simulink model "LongPRACH_sim"  (R2023b)
settings: Solver=FixedStepDiscrete  StartTime=0.0  StopTime=prach.SimulationTime  FixedStep=1  RelTol=1e-3  EnableMultiTasking=on
PreLoadFcn:
  | warning off Simulink:Commands:SetParamLinkChangeWarn
  | warning off Simulink:Commands:LoadMdlParameterizedLink
  | warning off Simulink:SL_SetParamLinkChangeWarn
  | warning off Simulink:SL_LoadMdlParameterizedLink
  | setup_LongPRACH;
InitFcn:
  | setup_LongPRACH;
StopFcn:
  | %prach_out_analysis;
  | prach_analysis
values from neighbouring files (symbols this model uses):
  prach = nrPRACHConfig('FrequencyRange','FR1','DuplexMode','TDD','ConfigurationIndex',config_idx,'SubcarrierSpacing',1.25,'SequenceIndex',ZCseq,          'PreambleIndex', cs_idx,'RBOffset',nRB,'ZeroCorrelationZone', N_cs, 'RestrictedSet','UnrestrictedSet', 'ActivePRACHSlot', 0 ,'FrequencyIndex', ii-1, 'TimeIndex',0,'NPRACHSlot',0)    [prach_gen_5g_toolbox.m]
undefined symbols (not defined in the file or in its folder): dpoly, value
libraries: DSPBAPrim x27, DSPBABase x7, dspsrcs4 x3, DSPBAUtilities x1, DSPBAControl x1, Lib_LongPRACH x1
Description:
  | This design example implements a long PRACH format-0 processing for NR - RU
settings Model: Creator=lrigby  LastModifiedBy=manjukri
settings SolverCC: AlgebraicLoopSolver=TrustRegion
settings DataIOCC: LimitDataPoints=on  SaveFormat=Array  SignalLoggingSaveFormat=ModelDataLogs  ReturnWorkspaceOutputs=off
settings OptimizationCC: ExpressionDepthLimit=2147483647  InitFltsAndDblsToZero=on  LifeSpan=inf
settings DebuggingCC: SaveWithParameterizedLinksMsg=none  UnderspecifiedInitializationDetection=Classic  MergeDetectMultiDrivingBlocksExec=none  SignalResolutionControl=TryResolveAllWithWarning  SolverPrmCheckMsg=warning  ParameterPrecisionLossMsg=none  UnconnectedInputMsg=warning  UnconnectedOutputMsg=warning  UnconnectedLineMsg=warning  StateNameClashWarn=warning  SFUnexpectedBacktrackingDiag=warning  SFNoUnconditionalDefaultTransitionDiag=warning  SFExecutionAtInitializationDiag=none  ArithmeticOperatorsInVariantConditions=warning
settings HardwareCC: ProdBitPerPointer=32  ProdBitPerSizeT=32  ProdBitPerPtrDiffT=32  ProdLargestAtomicFloat=None  ProdIntDivRoundTo=Undefined  ProdEndianess=Unspecified  ProdWordSize=32  ProdHWDeviceType=ASIC/FPGA  TargetBitPerLong=64  TargetBitPerPointer=64  TargetBitPerSizeT=64  TargetBitPerPtrDiffT=64  TargetLongLongMode=on  TargetIntDivRoundTo=Zero  TargetEndianess=LittleEndian  TargetWordSize=64  TargetHWDeviceType=MATLAB Host  ProdEqTarget=off
settings ModelReferenceCC: EnableRefExpFcnMdlSchedulingChecks=on  PropagateSignalLabelsOutOfModel=off
settings SFSimCC: SimUseLocalCustomCode=off  SimParseCustomCode=off  CustomCodeUndefinedFunction=UseInterfaceOnly
settings RTWCC: RTWUseLocalCustomCode=off  DLArmComputeVersion=19.05
settings CodeAppCC: StateflowObjectComments=on
settings GRTTargetCC: TargetFcnLib=ansi_tfl_tmw.mat  TargetLangStandard=C89/C90 (ANSI)  CombineOutputUpdateFcns=off  GRTInterface=on
settings ConfigComp: CovMetricSettings=dw  CovSaveCumulativeToWorkspaceVar=on  CovSaveSingleToWorkspaceVar=on  CovExternalEMLEnable=off  CovSFcnEnable=off

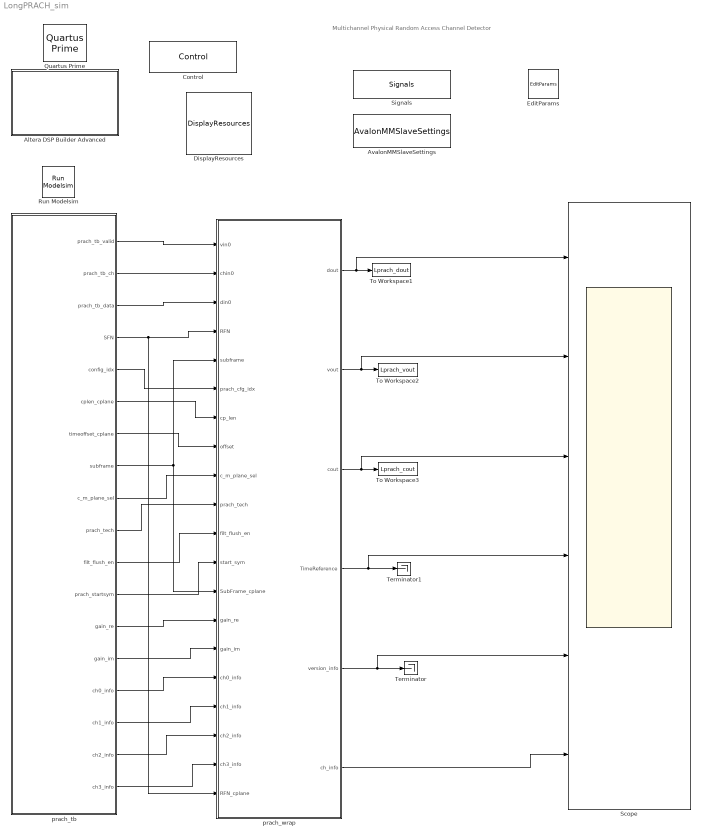
== system LongPRACH_sim ==
  note: Multichannel Physical Random
      | Access Channel Detector
  Altera DSP Builder Advanced : Subsystem  mask(DSP Builder Advanced Blockset Ignored Block){}
      settings: OpenFcn=web('http://www.altera.com', '-new');
      mask Display: image(imread('alteralogo.tif'));
  AvalonMMSlaveSettings : DSPBABase/AvalonMMSlaveSettings
  Control : DSPBABase/Control  generate=on  language=VHDL  destination=rtl  make_full_path=off  path_is_relative=on  autotestbench=on  signaldepth=2  coveragetestbench=off  logs=off  spacewidth=2  spacenum=1  addrwidth=10  datawidth=16  dataendian=Big Endian  hierarchicalnames=on  ramThresholdBits=-1  distRamThresholdBits=-1  mlabThresholdBits=-1  hardMultiplierThresholdLuts=-1  version=20090407  errorOnChanMismatch=1  errorOnGPIOMismatch=0  importModelsimResults=0  cycleAccurate=off  reinterpretCastMult=off  paramFile=LongPRACH_sim_params.xml
  DisplayResources : DSPBAUtilities/DisplayResources  mults=0  luts=0  memorybits=0
  EditParams : DSPBABase/EditParams  version=20090407
  Quartus Prime : DSPBABase/Quartus Prime  version=20090407
  Run Modelsim : DSPBABase/Run Modelsim  version=20090407
  Scope : Scope  NumInputPorts=6
  Signals : DSPBABase/Signals  clk=clk  freq=240  margin=0  rst=areset  rstactive=High  bus=bus  enbusclock=off  busfreq=491.52  bussync=off  version=20090407
  Terminator : Terminator
  Terminator1 : Terminator
  To Workspace1 : ToWorkspace  VariableName=Lprach_dout  SaveFormat=Timeseries  SampleTime=-1
  To Workspace2 : ToWorkspace  VariableName=Lprach_vout  SaveFormat=Timeseries  SampleTime=-1
  To Workspace3 : ToWorkspace  VariableName=Lprach_cout  SaveFormat=Timeseries  SampleTime=-1
  prach_tb : Subsystem
  prach_wrap : Subsystem
  wires:
  prach_wrap/3(cout) -> Scope/3, To Workspace3/1
  prach_tb/1(prach_tb_valid) -> prach_wrap/1(vin0)
  prach_wrap/2(vout) -> Scope/2, To Workspace2/1
  prach_tb/3(prach_tb_data) -> prach_wrap/3(din0)
  prach_tb/4(SFN) -> prach_wrap/20(RFN_cplane), prach_wrap/4(RFN)
  prach_tb/5(config_idx) -> prach_wrap/6(prach_cfg_idx)
  prach_tb/7(timeoffset_cplane) -> prach_wrap/8(offset)
  prach_tb/9(c_m_plane_sel) -> prach_wrap/9(c_m_plane_sel)
  prach_tb/8(subframe) -> prach_wrap/13(SubFrame_cplane), prach_wrap/5(subframe)
  prach_tb/2(prach_tb_ch) -> prach_wrap/2(chin0)
  prach_tb/6(cplen_cplane) -> prach_wrap/7(cp_len)
  prach_tb/10(prach_tech) -> prach_wrap/10(prach_tech)
  prach_tb/11(filt_flush_en) -> prach_wrap/11(filt_flush_en)
  prach_tb/12(prach_startsym) -> prach_wrap/12(start_sym)
  prach_wrap/1(dout) -> Scope/1, To Workspace1/1
  prach_tb/13(gain_re) -> prach_wrap/14(gain_re)
  prach_tb/14(gain_im) -> prach_wrap/15(gain_im)
  prach_wrap/5(version_info) -> Scope/5, Terminator/1
  prach_wrap/4(TimeReference) -> Scope/4, Terminator1/1
  prach_wrap/6(ch_info) -> Scope/6
  prach_tb/15(ch0_info) -> prach_wrap/16(ch0_info)
  prach_tb/16(ch1_info) -> prach_wrap/17(ch1_info)
  prach_tb/17(ch2_info) -> prach_wrap/18(ch2_info)
  prach_tb/18(ch3_info) -> prach_wrap/19(ch3_info)

== system LongPRACH_sim/Altera DSP Builder Advanced ==

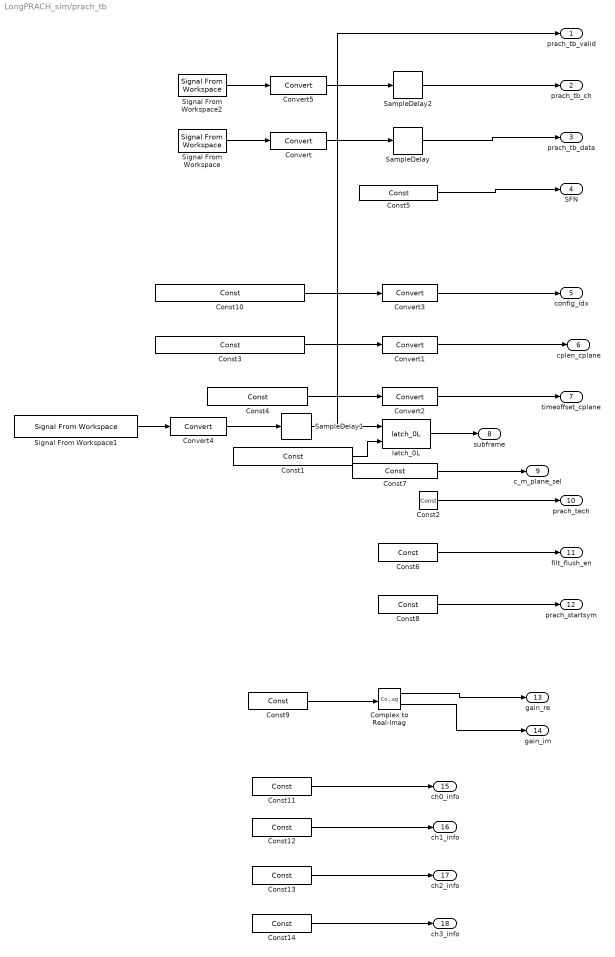
== system LongPRACH_sim/prach_tb ==
  Complex to Real-Imag : ComplexToRealImag
  Const1 : DSPBAPrim/Const  primtype=const  nInputs=0  nOutputs=1  omode=Specify via dialog  otype=uint(8)  scale=2^-0  rndmethod=Unbiased  factor=1  satmethod=Symmetric  shift_vec=[0 1 2 -1]  value=lprach_tb_in_local.subframe  inPortNames=['+'; '+';]  outPortNames=[' ']  dspbaimage=dspba_prim.svg  text=fprintf('%s', num2str(value));  style=Optimised  visibilities=8 + 1024  floatPrecision=float32_m23  warnSaturation=on  version=20211007  SampleTime=inf
  Const10 : DSPBAPrim/Const  primtype=const  nInputs=0  nOutputs=1  omode=Inherit via internal rule  otype=uint(8)  scale=2^-0  rndmethod=Unbiased  factor=1  satmethod=Symmetric  shift_vec=[0 1 2 -1]  value=lprach_tb_exp_out_local.prach.ConfigIndex  inPortNames=['+'; '+';]  outPortNames=[' ']  dspbaimage=dspba_prim.svg  text=fprintf('%s', num2str(value));  style=Optimised  visibilities=8 + 1024  floatPrecision=float32_m23  warnSaturation=on  version=20211007  SampleTime=inf
  Const11 : DSPBAPrim/Const  primtype=const  nInputs=0  nOutputs=1  omode=Specify via dialog  otype=ufix(16)  scale=0  rndmethod=Unbiased  factor=1  satmethod=Symmetric  shift_vec=[0 1 2 -1]  value=0  inPortNames=['+'; '+';]  outPortNames=[' ']  dspbaimage=dspba_prim.svg  text=fprintf('%s', num2str(value));  style=Optimised  visibilities=8 + 1024  floatPrecision=float32_m23  warnSaturation=on  version=20211007  SampleTime=inf
  Const12 : DSPBAPrim/Const  primtype=const  nInputs=0  nOutputs=1  omode=Specify via dialog  otype=ufix(16)  scale=0  rndmethod=Unbiased  factor=1  satmethod=Symmetric  shift_vec=[0 1 2 -1]  value=1  inPortNames=['+'; '+';]  outPortNames=[' ']  dspbaimage=dspba_prim.svg  text=fprintf('%s', num2str(value));  style=Optimised  visibilities=8 + 1024  floatPrecision=float32_m23  warnSaturation=on  version=20211007  SampleTime=inf
  Const13 : DSPBAPrim/Const  primtype=const  nInputs=0  nOutputs=1  omode=Specify via dialog  otype=ufix(16)  scale=0  rndmethod=Unbiased  factor=1  satmethod=Symmetric  shift_vec=[0 1 2 -1]  value=2  inPortNames=['+'; '+';]  outPortNames=[' ']  dspbaimage=dspba_prim.svg  text=fprintf('%s', num2str(value));  style=Optimised  visibilities=8 + 1024  floatPrecision=float32_m23  warnSaturation=on  version=20211007  SampleTime=inf
  Const14 : DSPBAPrim/Const  primtype=const  nInputs=0  nOutputs=1  omode=Specify via dialog  otype=ufix(16)  scale=0  rndmethod=Unbiased  factor=1  satmethod=Symmetric  shift_vec=[0 1 2 -1]  value=3  inPortNames=['+'; '+';]  outPortNames=[' ']  dspbaimage=dspba_prim.svg  text=fprintf('%s', num2str(value));  style=Optimised  visibilities=8 + 1024  floatPrecision=float32_m23  warnSaturation=on  version=20211007  SampleTime=inf
  Const2 : DSPBAPrim/Const  primtype=const  nInputs=0  nOutputs=1  omode=boolean  otype=uint(8)  scale=2^-0  rndmethod=Unbiased  factor=1  satmethod=Symmetric  shift_vec=[0 1 2 -1]  value=lprach_tb_in_local.prach_tech  inPortNames=['+'; '+';]  outPortNames=[' ']  dspbaimage=dspba_prim.svg  text=fprintf('%s', num2str(value));  style=Optimised  visibilities=8 + 1024  floatPrecision=float32_m23  warnSaturation=on  version=20211007  SampleTime=inf
  Const3 : DSPBAPrim/Const  primtype=const  nInputs=0  nOutputs=1  omode=Inherit via internal rule  otype=uint(8)  scale=2^-0  rndmethod=Unbiased  factor=1  satmethod=Symmetric  shift_vec=[0 1 2 -1]  value=lprach_tb_in_local.cp_len  inPortNames=['+'; '+';]  outPortNames=[' ']  dspbaimage=dspba_prim.svg  text=fprintf('%s', num2str(value));  style=Optimised  visibilities=8 + 1024  floatPrecision=float32_m23  warnSaturation=on  version=20211007  SampleTime=inf
  Const4 : DSPBAPrim/Const  primtype=const  nInputs=0  nOutputs=1  omode=Inherit via internal rule  otype=uint(8)  scale=2^-0  rndmethod=Unbiased  factor=1  satmethod=Symmetric  shift_vec=[0 1 2 -1]  value=lprach_tb_in_local.Timeoffset_input  inPortNames=['+'; '+';]  outPortNames=[' ']  dspbaimage=dspba_prim.svg  text=fprintf('%s', num2str(value));  style=Optimised  visibilities=8 + 1024  floatPrecision=float32_m23  warnSaturation=on  version=20211007  SampleTime=inf
  Const5 : DSPBAPrim/Const  primtype=const  nInputs=0  nOutputs=1  omode=Specify via dialog  otype=uint(12)  scale=2^-0  rndmethod=Unbiased  factor=1  satmethod=Symmetric  shift_vec=[0 1 2 -1]  value=lprach_tb_in_local.SFN  inPortNames=['+'; '+';]  outPortNames=[' ']  dspbaimage=dspba_prim.svg  text=fprintf('%s', num2str(value));  style=Optimised  visibilities=8 + 1024  floatPrecision=float32_m23  warnSaturation=on  version=20211007  SampleTime=inf
  Const6 : DSPBAPrim/Const  primtype=const  nInputs=0  nOutputs=1  omode=boolean  otype=uint(8)  scale=2^-0  rndmethod=Unbiased  factor=1  satmethod=Symmetric  shift_vec=[0 1 2 -1]  value=filt_flush_enable  inPortNames=['+'; '+';]  outPortNames=[' ']  dspbaimage=dspba_prim.svg  text=fprintf('%s', num2str(value));  style=Optimised  visibilities=8 + 1024  floatPrecision=float32_m23  warnSaturation=on  version=20211007  SampleTime=inf
  Const7 : DSPBAPrim/Const  primtype=const  nInputs=0  nOutputs=1  omode=boolean  otype=uint(8)  scale=2^-0  rndmethod=Unbiased  factor=1  satmethod=Symmetric  shift_vec=[0 1 2 -1]  value=lprach_tb_in_local.c_m_plane_sel  inPortNames=['+'; '+';]  outPortNames=[' ']  dspbaimage=dspba_prim.svg  text=fprintf('%s', num2str(value));  style=Optimised  visibilities=8 + 1024  floatPrecision=float32_m23  warnSaturation=on  version=20211007  SampleTime=inf
  Const8 : DSPBAPrim/Const  primtype=const  nInputs=0  nOutputs=1  omode=Specify via dialog  otype=ufix(4)  scale=0  rndmethod=Unbiased  factor=1  satmethod=Symmetric  shift_vec=[0 1 2 -1]  value=lprach_tb_in_local.prach.StartSym  inPortNames=['+'; '+';]  outPortNames=[' ']  dspbaimage=dspba_prim.svg  text=fprintf('%s', num2str(value));  style=Optimised  visibilities=8 + 1024  floatPrecision=float32_m23  warnSaturation=on  version=20211007  SampleTime=inf
  Const9 : DSPBAPrim/Const  primtype=const  nInputs=0  nOutputs=1  omode=Specify via dialog  otype=fixdt(0,16,14)  scale=0  rndmethod=Unbiased  factor=1  satmethod=Symmetric  shift_vec=[0 1 2 -1]  value=lprach_tb_in.gain  inPortNames=['+'; '+';]  outPortNames=[' ']  dspbaimage=dspba_prim.svg  text=fprintf('%s', num2str(value));  style=Optimised  visibilities=8 + 1024  floatPrecision=float32_m23  warnSaturation=on  version=20211007  SampleTime=inf
  Convert : DSPBAPrim/Convert  primtype=convert  nInputs=1  nOutputs=1  omode=Specify via dialog  otype=sfix(16)  scale=2^-14  rndmethod=Biased  factor=1  satmethod=None  shift_vec=[0 1 2 -1]  value=round([0:255]/17)  inPortNames=[' '; ' ';]  outPortNames=[' '; 'c']  dspbaimage=dspba_prim_wide.svg  text=fprintf('convert');  style=Optimised  visibilities=8+64+256+2^17  clipdetect=off  floatPrecision=float32_m23  advOptions=[]  version=20211007
  Convert1 : DSPBAPrim/Convert  primtype=convert  nInputs=1  nOutputs=1  omode=Specify via dialog  otype=ufix(21)  scale=2^0  rndmethod=Biased  factor=1  satmethod=None  shift_vec=[0 1 2 -1]  value=round([0:255]/17)  inPortNames=[' '; ' ';]  outPortNames=[' '; 'c']  dspbaimage=dspba_prim_wide.svg  text=fprintf('convert');  style=Optimised  visibilities=8+64+256+2^17  clipdetect=off  floatPrecision=float32_m23  advOptions=[]  version=20211007
  Convert2 : DSPBAPrim/Convert  primtype=convert  nInputs=1  nOutputs=1  omode=Specify via dialog  otype=ufix(21)  scale=2^0  rndmethod=Biased  factor=1  satmethod=None  shift_vec=[0 1 2 -1]  value=round([0:255]/17)  inPortNames=[' '; ' ';]  outPortNames=[' '; 'c']  dspbaimage=dspba_prim_wide.svg  text=fprintf('convert');  style=Optimised  visibilities=8+64+256+2^17  clipdetect=off  floatPrecision=float32_m23  advOptions=[]  version=20211007
  Convert3 : DSPBAPrim/Convert  primtype=convert  nInputs=1  nOutputs=1  omode=Specify via dialog  otype=ufix(16)  scale=2^0  rndmethod=Biased  factor=1  satmethod=None  shift_vec=[0 1 2 -1]  value=round([0:255]/17)  inPortNames=[' '; ' ';]  outPortNames=[' '; 'c']  dspbaimage=dspba_prim_wide.svg  text=fprintf('convert');  style=Optimised  visibilities=8+64+256+2^17  clipdetect=off  floatPrecision=float32_m23  advOptions=[]  version=20211007
  Convert4 : DSPBAPrim/Convert  primtype=convert  nInputs=1  nOutputs=1  omode=boolean  otype=sfix(16)  scale=2^-14  rndmethod=Biased  factor=1  satmethod=None  shift_vec=[0 1 2 -1]  value=round([0:255]/17)  inPortNames=[' '; ' ';]  outPortNames=[' '; 'c']  dspbaimage=dspba_prim_wide.svg  text=fprintf('convert');  style=Optimised  visibilities=8+64+256+2^17  clipdetect=off  floatPrecision=float32_m23  advOptions=[]  version=20211007
  Convert5 : DSPBAPrim/Convert  primtype=convert  nInputs=1  nOutputs=1  omode=Specify via dialog  otype=fixdt(0,8,0)  scale=0  rndmethod=Biased  factor=1  satmethod=None  shift_vec=[0 1 2 -1]  value=round([0:255]/17)  inPortNames=[' '; ' ';]  outPortNames=[' '; 'c']  dspbaimage=dspba_prim_wide.svg  text=fprintf('convert');  style=Optimised  visibilities=8+64+256+2^17  clipdetect=off  floatPrecision=float32_m23  advOptions=[]  version=20211007
  SampleDelay : DSPBAPrim/SampleDelay  primtype=sampdelay  nInputs=1  nOutputs=1  omode=Inherit via internal rule  otype=sfix(16)  scale=2^-15  rndmethod=Unbiased  factor=1  satmethod=Symmetric  shift_vec=[0 1 2 -1]  floatPrecision=float32_m23  value=100  inPortNames=[' '; ' ';]  outPortNames=[' ']  dspbaimage=dspba_prim.svg  text=dpoly(1, eye(1,value+1), 'z')  style=Optimised  visibilities=8 + 1024 + 2^17 + 2^18  flexible=off  slackgroup=0  augmented=0  version=20211007  advOptions=[]
  SampleDelay1 : DSPBAPrim/SampleDelay  primtype=sampdelay  nInputs=1  nOutputs=1  omode=Inherit via internal rule  otype=sfix(16)  scale=2^-15  rndmethod=Unbiased  factor=1  satmethod=Symmetric  shift_vec=[0 1 2 -1]  floatPrecision=float32_m23  value=100  inPortNames=[' '; ' ';]  outPortNames=[' ']  dspbaimage=dspba_prim.svg  text=dpoly(1, eye(1,value+1), 'z')  style=Optimised  visibilities=8 + 1024 + 2^17 + 2^18  flexible=off  slackgroup=0  augmented=0  version=20211007  advOptions=[]
  SampleDelay2 : DSPBAPrim/SampleDelay  primtype=sampdelay  nInputs=1  nOutputs=1  omode=Inherit via internal rule  otype=sfix(16)  scale=2^-15  rndmethod=Unbiased  factor=1  satmethod=Symmetric  shift_vec=[0 1 2 -1]  floatPrecision=float32_m23  value=100  inPortNames=[' '; ' ';]  outPortNames=[' ']  dspbaimage=dspba_prim.svg  text=dpoly(1, eye(1,value+1), 'z')  style=Optimised  visibilities=8 + 1024 + 2^17 + 2^18  flexible=off  slackgroup=0  augmented=0  version=20211007  advOptions=[]
  Signal From Workspace : dspsrcs4/Signal From Workspace  X=lprach_tb_in.Prach_tb_data  Ts=prach.SampleTime  nsamps=1  OutputAfterFinalValue=Cyclic repetition  ignoreOrWarnInputAndFrameLengths=off  OutputFrames=off
  Signal From Workspace1 : dspsrcs4/Signal From Workspace  X=lprach_tb_in_local.Prach_tb_valid  Ts=prach.SampleTime  nsamps=1  OutputAfterFinalValue=Cyclic repetition  ignoreOrWarnInputAndFrameLengths=off  OutputFrames=off
  Signal From Workspace2 : dspsrcs4/Signal From Workspace  X=lprach_tb_in.Prach_tb_ch  Ts=prach.SampleTime  nsamps=1  OutputAfterFinalValue=Cyclic repetition  ignoreOrWarnInputAndFrameLengths=off  OutputFrames=off
  latch_0L : DSPBAControl/latch_0L
  prach_tb_valid : Outport
  prach_tb_ch : Outport  Port=2
  prach_tb_data : Outport  Port=3
  SFN : Outport  Port=4
  config_idx : Outport  Port=5
  cplen_cplane : Outport  Port=6
  timeoffset_cplane : Outport  Port=7
  subframe : Outport  Port=8
  c_m_plane_sel : Outport  Port=9
  prach_tech : Outport  Port=10
  filt_flush_en : Outport  Port=11
  prach_startsym : Outport  Port=12
  gain_re : Outport  Port=13
  gain_im : Outport  Port=14
  ch0_info : Outport  Port=15
  ch1_info : Outport  Port=16
  ch2_info : Outport  Port=17
  ch3_info : Outport  Port=18
  wires:
  Const8/1 -> prach_startsym/1
  Convert/1 -> SampleDelay/1
  Const1/1 -> latch_0L/2
  Const7/1 -> c_m_plane_sel/1
  Signal From Workspace1/1 -> Convert4/1
  Const2/1 -> prach_tech/1
  Convert1/1 -> cplen_cplane/1
  SampleDelay1/1 -> prach_tb_valid/1, latch_0L/1
  Convert2/1 -> timeoffset_cplane/1
  Convert3/1 -> config_idx/1
  Convert5/1 -> SampleDelay2/1
  SampleDelay/1 -> prach_tb_data/1
  Const4/1 -> Convert2/1
  Signal From Workspace2/1 -> Convert5/1
  SampleDelay2/1 -> prach_tb_ch/1
  Const3/1 -> Convert1/1
  Const5/1 -> SFN/1
  Const6/1 -> filt_flush_en/1
  Signal From Workspace/1 -> Convert/1
  latch_0L/1 -> subframe/1
  Convert4/1 -> SampleDelay1/1
  Const10/1 -> Convert3/1
  Const9/1 -> Complex to Real-Imag/1
  Complex to Real-Imag/1 -> gain_re/1
  Complex to Real-Imag/2 -> gain_im/1
  Const11/1 -> ch0_info/1
  Const12/1 -> ch1_info/1
  Const13/1 -> ch2_info/1
  Const14/1 -> ch3_info/1

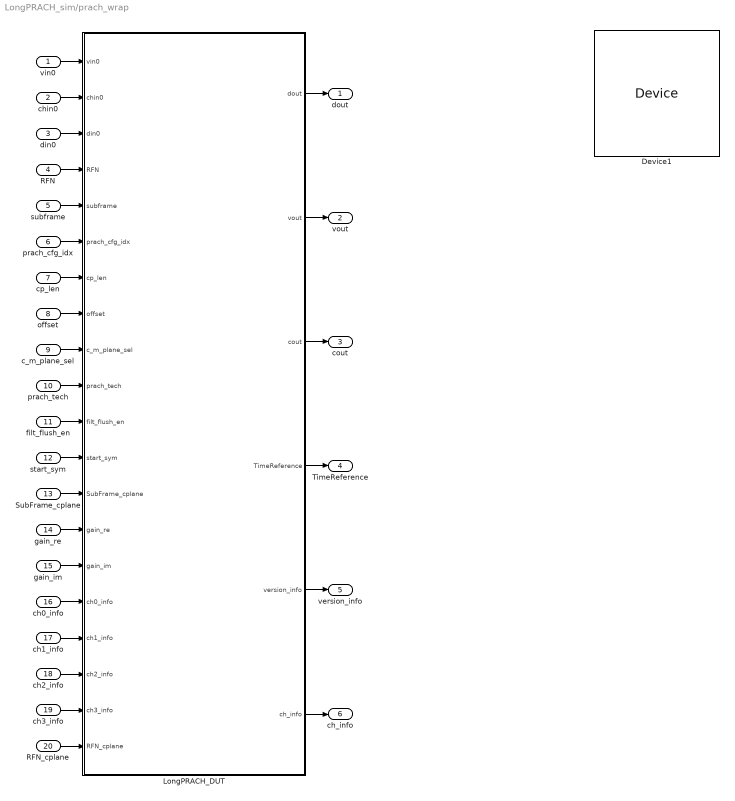
== system LongPRACH_sim/prach_wrap ==
  vin0 : Inport
  chin0 : Inport  Port=2
  din0 : Inport  Port=3
  RFN : Inport  Port=4
  subframe : Inport  Port=5
  prach_cfg_idx : Inport  Port=6
  cp_len : Inport  Port=7
  offset : Inport  Port=8
  c_m_plane_sel : Inport  Port=9
  prach_tech : Inport  Port=10
  filt_flush_en : Inport  Port=11
  start_sym : Inport  Port=12
  SubFrame_cplane : Inport  Port=13
  gain_re : Inport  Port=14
  gain_im : Inport  Port=15
  ch0_info : Inport  Port=16
  ch1_info : Inport  Port=17
  ch2_info : Inport  Port=18
  ch3_info : Inport  Port=19
  RFN_cplane : Inport  Port=20
  Device1 : DSPBABase/Device  family=Arria 10  stratix4device=Stratix IV E  hardcopy4device=HardCopy IV E  stratix5device=Stratix V GX  device=AUTO  speed=1_H1  stratixSpeed=-5  stratix2Speed=-3  stratix3Speed=-2  stratix4gxSpeed=-2  stratix4gtSpeed=-1  cyclone2Speed=-6  cyclone3Speed=-7  arria2Speed=-4  cyclone4eSpeed=-8  stratix5Speed=-3  arria5Speed=-4  arriaSpeed=-6  cyclone3lsSpeed=-7  cyclone5Speed=-6  arria2gzSpeed=-3  nightFurySpeed=-2  ecp2Speed=-7  hardcopycompat=off  version=20140217  max10flashmode=off  max10nomeminit=off
  LongPRACH_DUT : Subsystem
  dout : Outport
  vout : Outport  Port=2
  cout : Outport  Port=3
  TimeReference : Outport  Port=4
  version_info : Outport  Port=5
  ch_info : Outport  Port=6
  wires:
  LongPRACH_DUT/6(ch_info) -> ch_info/1
  LongPRACH_DUT/4(TimeReference) -> TimeReference/1
  LongPRACH_DUT/2(vout) -> vout/1
  LongPRACH_DUT/1(dout) -> dout/1
  ch2_info/1 -> LongPRACH_DUT/18(ch2_info)
  ch1_info/1 -> LongPRACH_DUT/17(ch1_info)
  ch0_info/1 -> LongPRACH_DUT/16(ch0_info)
  LongPRACH_DUT/3(cout) -> cout/1
  gain_im/1 -> LongPRACH_DUT/15(gain_im)
  vin0/1 -> LongPRACH_DUT/1(vin0)
  filt_flush_en/1 -> LongPRACH_DUT/11(filt_flush_en)
  chin0/1 -> LongPRACH_DUT/2(chin0)
  din0/1 -> LongPRACH_DUT/3(din0)
  RFN/1 -> LongPRACH_DUT/4(RFN)
  LongPRACH_DUT/5(version_info) -> version_info/1
  start_sym/1 -> LongPRACH_DUT/12(start_sym)
  subframe/1 -> LongPRACH_DUT/5(subframe)
  ch3_info/1 -> LongPRACH_DUT/19(ch3_info)
  prach_cfg_idx/1 -> LongPRACH_DUT/6(prach_cfg_idx)
  offset/1 -> LongPRACH_DUT/8(offset)
  prach_tech/1 -> LongPRACH_DUT/10(prach_tech)
  cp_len/1 -> LongPRACH_DUT/7(cp_len)
  c_m_plane_sel/1 -> LongPRACH_DUT/9(c_m_plane_sel)
  gain_re/1 -> LongPRACH_DUT/14(gain_re)
  SubFrame_cplane/1 -> LongPRACH_DUT/13(SubFrame_cplane)
  RFN_cplane/1 -> LongPRACH_DUT/20(RFN_cplane)

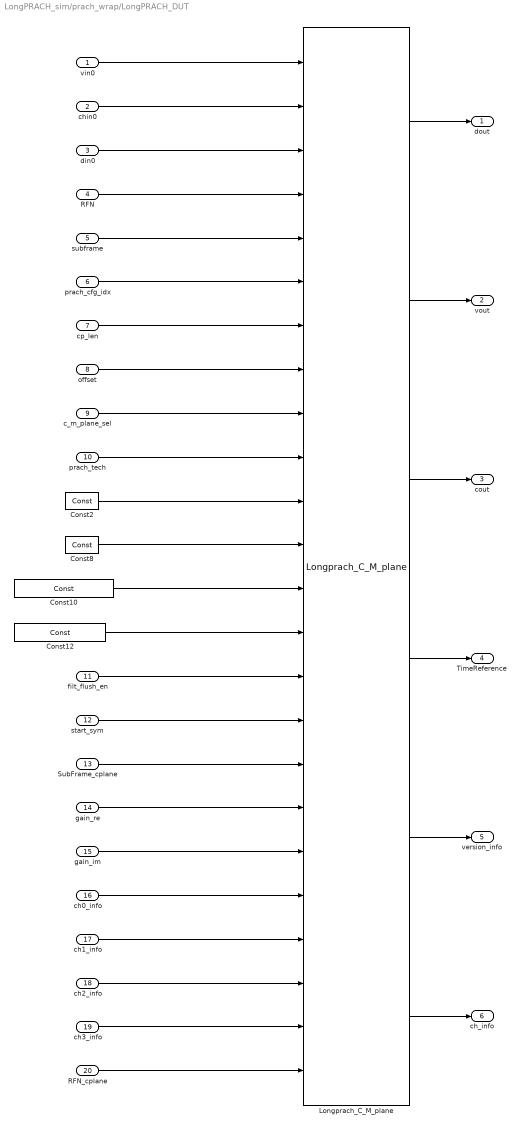
== system LongPRACH_sim/prach_wrap/LongPRACH_DUT ==
  vin0 : Inport
  chin0 : Inport  Port=2
  din0 : Inport  Port=3
  RFN : Inport  Port=4
  subframe : Inport  Port=5
  prach_cfg_idx : Inport  Port=6
  cp_len : Inport  Port=7
  offset : Inport  Port=8
  c_m_plane_sel : Inport  Port=9
  prach_tech : Inport  Port=10
  filt_flush_en : Inport  Port=11
  start_sym : Inport  Port=12
  SubFrame_cplane : Inport  Port=13
  gain_re : Inport  Port=14
  gain_im : Inport  Port=15
  ch0_info : Inport  Port=16
  ch1_info : Inport  Port=17
  ch2_info : Inport  Port=18
  ch3_info : Inport  Port=19
  RFN_cplane : Inport  Port=20
  Const10 : DSPBAPrim/Const  primtype=const  nInputs=0  nOutputs=1  omode=Inherit via internal rule  otype=uint(8)  scale=2^-0  rndmethod=Unbiased  factor=1  satmethod=Symmetric  shift_vec=[0 1 2 -1]  value=prach.SCstart-1  inPortNames=['+'; '+';]  outPortNames=[' ']  dspbaimage=dspba_prim.svg  text=fprintf('%s', num2str(value));  style=Optimised  visibilities=8 + 1024  floatPrecision=float32_m23  warnSaturation=on  version=20211007  SampleTime=inf
  Const12 : DSPBAPrim/Const  primtype=const  nInputs=0  nOutputs=1  omode=Inherit via internal rule  otype=uint(8)  scale=2^-0  rndmethod=Unbiased  factor=1  satmethod=Symmetric  shift_vec=[0 1 2 -1]  value=prach.SCend  inPortNames=['+'; '+';]  outPortNames=[' ']  dspbaimage=dspba_prim.svg  text=fprintf('%s', num2str(value));  style=Optimised  visibilities=8 + 1024  floatPrecision=float32_m23  warnSaturation=on  version=20211007  SampleTime=inf
  Const2 : DSPBAPrim/Const  primtype=const  nInputs=0  nOutputs=1  omode=Inherit via internal rule  otype=uint(8)  scale=2^-0  rndmethod=Unbiased  factor=1  satmethod=Symmetric  shift_vec=[0 1 2 -1]  value=50688  inPortNames=['+'; '+';]  outPortNames=[' ']  dspbaimage=dspba_prim.svg  text=fprintf('%s', num2str(value));  style=Optimised  visibilities=8 + 1024  floatPrecision=float32_m23  warnSaturation=on  version=20211007  SampleTime=inf
  Const8 : DSPBAPrim/Const  primtype=const  nInputs=0  nOutputs=1  omode=Inherit via internal rule  otype=uint(8)  scale=2^-0  rndmethod=Unbiased  factor=1  satmethod=Symmetric  shift_vec=[0 1 2 -1]  value=443904  inPortNames=['+'; '+';]  outPortNames=[' ']  dspbaimage=dspba_prim.svg  text=fprintf('%s', num2str(value));  style=Optimised  visibilities=8 + 1024  floatPrecision=float32_m23  warnSaturation=on  version=20211007  SampleTime=inf
  Longprach_C_M_plane : Lib_LongPRACH/Longprach_C_M_plane  AxCdelay=60  FFT_frac_scaling=8  gain_out_frac=13
      link override LongPRACH_core/DECIMATION1/Stage1/Filt_DEC_by_3_stage1/DecimatingFIR1: latency=25
      link override LongPRACH_core/DECIMATION1/Stage1/Filt_DEC_by_3_stage1/DecimatingFIR2: latency=25
      link override LongPRACH_core/DECIMATION1/Stage1/Filt_DEC_by_3_stage1/Scale: latency=2
      link override LongPRACH_core/DECIMATION1/Stage1/Filt_DEC_by_3_stage1/Scale1: latency=2
      link override LongPRACH_core/DECIMATION1/Stage2/Filt_DEC_by_2_stage2/DecimatingFIR: latency=29
      link override LongPRACH_core/DECIMATION1/Stage2/Filt_DEC_by_2_stage2/DecimatingFIR1: latency=29
      link override LongPRACH_core/DECIMATION1/Stage2/Filt_DEC_by_2_stage2/Scale: latency=2
      link override LongPRACH_core/DECIMATION1/Stage2/Filt_DEC_by_2_stage2/Scale1: latency=2
      link override LongPRACH_core/DECIMATION1/Stage3/Filt_DEC_by_2_stage3/DecimatingFIR: latency=47
      link override LongPRACH_core/DECIMATION1/Stage3/Filt_DEC_by_2_stage3/DecimatingFIR1: latency=47
      link override LongPRACH_core/DECIMATION1/Stage3/Filt_DEC_by_2_stage3/Scale: latency=2
      link override LongPRACH_core/DECIMATION1/Stage3/Filt_DEC_by_2_stage3/Scale1: latency=2
      link override LongPRACH_core/DECIMATION1/Stage5/Filt_DEC_by_2_stage5/DecimatingFIR: latency=47
      link override LongPRACH_core/DECIMATION1/Stage5/Filt_DEC_by_2_stage5/DecimatingFIR1: latency=47
      link override LongPRACH_core/DECIMATION1/Stage5/Filt_DEC_by_2_stage5/Scale: latency=2
      link override LongPRACH_core/DECIMATION1/Stage5/Filt_DEC_by_2_stage5/Scale1: latency=2
      link override LongPRACH_core/DECIMATION1/Stage6/Filt_DEC_by_2_stage6/DecimatingFIR: latency=183
      link override LongPRACH_core/DECIMATION1/Stage6/Filt_DEC_by_2_stage6/DecimatingFIR1: latency=183
      link override LongPRACH_core/DECIMATION1/Stage6/Filt_DEC_by_2_stage6/Scale: latency=3
      link override LongPRACH_core/DECIMATION1/Stage6/Filt_DEC_by_2_stage6/Scale1: latency=3
      link override LongPRACH_core/DECIMATION1/stage4/Filt_DEC_by_2_stage4/DecimatingFIR: latency=55
      link override LongPRACH_core/DECIMATION1/stage4/Filt_DEC_by_2_stage4/DecimatingFIR1: latency=55
      link override LongPRACH_core/DECIMATION1/stage4/Filt_DEC_by_2_stage4/Scale: latency=2
      link override LongPRACH_core/DECIMATION1/stage4/Filt_DEC_by_2_stage4/Scale1: latency=2
      link override LongPRACH_core/S2B_FFT/FFT1/ChannelOut1: latency=51
      link override LongPRACH_core/S2B_FFT/S2B/ChannelOut: latency=7
      link override LongPRACH_core/S2B_FFT/gain/ChannelOut: latency=8
      link override MUX_ConfigId/ChannelIn: dataSignals=15
      link override MUX_ConfigId/ChannelOut: latency=23
  dout : Outport
  vout : Outport  Port=2
  cout : Outport  Port=3
  TimeReference : Outport  Port=4
  version_info : Outport  Port=5
  ch_info : Outport  Port=6
  wires:
  Longprach_C_M_plane/6 -> ch_info/1
  offset/1 -> Longprach_C_M_plane/8
  Const10/1 -> Longprach_C_M_plane/13
  vin0/1 -> Longprach_C_M_plane/1
  ch1_info/1 -> Longprach_C_M_plane/21
  RFN_cplane/1 -> Longprach_C_M_plane/24
  Const2/1 -> Longprach_C_M_plane/11
  c_m_plane_sel/1 -> Longprach_C_M_plane/9
  din0/1 -> Longprach_C_M_plane/3
  gain_re/1 -> Longprach_C_M_plane/18
  Const8/1 -> Longprach_C_M_plane/12
  prach_cfg_idx/1 -> Longprach_C_M_plane/6
  prach_tech/1 -> Longprach_C_M_plane/10
  Longprach_C_M_plane/4 -> TimeReference/1
  RFN/1 -> Longprach_C_M_plane/4
  chin0/1 -> Longprach_C_M_plane/2
  subframe/1 -> Longprach_C_M_plane/5
  Const12/1 -> Longprach_C_M_plane/14
  filt_flush_en/1 -> Longprach_C_M_plane/15
  start_sym/1 -> Longprach_C_M_plane/16
  ch0_info/1 -> Longprach_C_M_plane/20
  cp_len/1 -> Longprach_C_M_plane/7
  SubFrame_cplane/1 -> Longprach_C_M_plane/17
  gain_im/1 -> Longprach_C_M_plane/19
  Longprach_C_M_plane/3 -> cout/1
  ch2_info/1 -> Longprach_C_M_plane/22
  Longprach_C_M_plane/5 -> version_info/1
  ch3_info/1 -> Longprach_C_M_plane/23
  Longprach_C_M_plane/1 -> dout/1
  Longprach_C_M_plane/2 -> vout/1
